simulink library "sm_rollerV_lib_underc_i1u2l7"  (R2026a)
settings: Solver=VariableStepAuto
undefined symbols (not defined in the file): Excv, L1, L2, L3, L4, L5, L6, L7, L8, L9, Left, P1, P2, P3, P4, P5, P6, P7, P8, P9, Right, shoe_w, X, Y, Z
libraries: sm_rollerV_lib_underc_elem x36, sm_lib x27, nesl_utility x20, sm_rollerV_lib_terrain_contact_belem x9, sm_trackV_lib_chain_underc_elem x8, fl_lib x4, sm_trackV_lib_frame_i1u2l7 x2
(part 2 of 3)

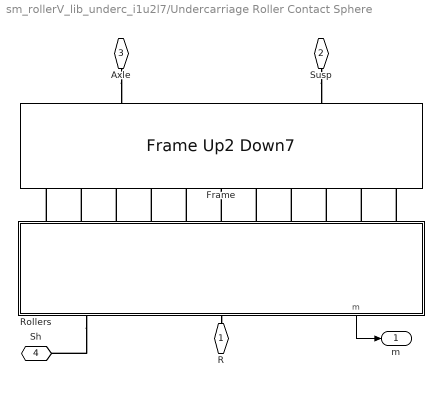
== system sm_rollerV_lib_underc_i1u2l7/Undercarriage Roller Contact Sphere ==
  Frame : sm_trackV_lib_frame_i1u2l7/Frame Up2 Down7  popup_leftOrRight=Right  roller_upper_x=roller_upper_x  roller_lower_x=roller_lower_x  idler_x=idler_x  axle_x=axle_x  roller_upper_y=roller_upper_y  roller_lower_y=roller_lower_y  idler_y=idler_y  axle_y=axle_y  frame_cg_offset=frame_cg_offset  frame_mass=frame_mass  frame_moi=frame_moi  frame_poi=frame_poi  frame_susp_offset=frame_susp_offset
  Rollers : Subsystem  mask(Rollers with Ground Contact (Spheres)){sprk_xc=sprk_xc, sprk_len=sprk_len, sprk_rho=sprk_rho, sprk_clr=sprk_clr, sprk_opc=sprk_opc, sprk_contact_geo_clr=sprk_contact_geo_clr, sprk_contact_geo_opc=sprk_contact_geo_opc, idler_rad=idler_rad, idler_len=idler_len, idler_rho=idler_rho, idler_clr=idler_clr, idler_opc=idler_opc, idler_contact_geo_clr=idler_contact_geo_clr, idler_contact_geo_opc=idler_contact_geo_opc, roller_upper_len=roller_upper_len, roller_upper_rad=roller_upper_rad, roller_upper_rho=roller_upper_rho, roller_upper_clr=roller_upper_clr, roller_upper_opc=roller_upper_opc, roller_upper_contgeo_clr=roller_upper_contgeo_clr, roller_upper_contgeo_opc=roller_upper_contgeo_opc, roller_lower_len=roller_lower_len, roller_lower_rad=roller_lower_rad, roller_lower_rho=roller_lower_rho, roller_lower_clr=roller_lower_clr, roller_lower_opc=roller_lower_opc, roller_lower_contgeo_clr=roller_lower_contgeo_clr, roller_lower_contgeo_opc=roller_lower_contgeo_opc, tensioner_cyl_rad=tensioner_cyl_rad, tensioner_cyl_len=tensioner_cyl_len, tensioner_cyl_rho=tensioner_cyl_rho, tensioner_cyl_clr=tensioner_cyl_clr, tensioner_cyl_opc=tensioner_cyl_opc, tensioner_pist_rad=tensioner_pist_rad, tensioner_pist_len=tensioner_pist_len, tensioner_pist_rho=tensioner_pist_rho, tensioner_pist_clr=tensioner_pist_clr, tensioner_pist_opc=tensioner_pist_opc, tensioner_br_length=tensioner_br_length, tensioner_br_width=tensioner_br_width, tensioner_br_height=tensioner_br_height, tensioner_br_thk=tensioner_br_thk, tensioner_br_rho=tensioner_br_rho, tensioner_br_clr=tensioner_br_clr, tensioner_br_opc=tensioner_br_opc, idler_max_ext=idler_max_ext, sprk_rolling_rad=sprk_rolling_rad, idler_rolling_rad=idler_rolling_rad, roller_lower_rolling_rad=roller_lower_rolling_rad, shoe_w=shoe_w, popup_sense_roller=Actuator Torque}
      mask prompts: sprk_xc "Extrusion Data [x y] (m)"; sprk_len "Length (m)"; sprk_rho "Density (kg/m^3)"; sprk_clr "Color [R G B] (0-1)"; sprk_opc "Opacity (0-1)"; sprk_contact_geo_clr "Color [R G B] (0-1)"; sprk_contact_geo_opc "Opacity (0-1)"; idler_rad "Radius (m)"; idler_len "Length(m)"; idler_rho "Density (kg/m^3)"; idler_clr "Color [R G B] (0-1)"; idler_opc "Opacity (0-1)"; idler_contact_geo_clr "Color [R G B] (0-1)"; idler_contact_geo_opc "Opacity (0-1)"; roller_upper_len "Length (m)"; roller_upper_rad "Radius (m)"; roller_upper_rho "Density (kg/m^3)"; roller_upper_clr "Color [R G B] (0-1)"; roller_upper_opc "Opacity (0-1)"; roller_upper_contgeo_clr "Color [R G B] (0-1)"; roller_upper_contgeo_opc "Opacity (0-1)"; roller_lower_len "Length (m)"; roller_lower_rad "Radius (m)"; roller_lower_rho "Density (kg/m^3)"; roller_lower_clr "Color [R G B] (0-1)"; roller_lower_opc "Opacity (0-1)"; roller_lower_contgeo_clr "Color [R G B] (0-1)"; roller_lower_contgeo_opc "Opacity (0-1)"; tensioner_cyl_rad "Radius (m)"; tensioner_cyl_len "Length (m)"; tensioner_cyl_rho "Density (kg/m^3)"; tensioner_cyl_clr "Color [R G B] (0-1)"; tensioner_cyl_opc "Opacity (0-1)"; tensioner_pist_rad "Radius (m)"; tensioner_pist_len "Length (m)"; tensioner_pist_rho "Density (kg/m^3)"; tensioner_pist_clr "Color [R G B] (0-1)"; tensioner_pist_opc "Opacity (0.1)"; tensioner_br_length "Length (m)"; tensioner_br_width "Width (m)"; tensioner_br_height "Height (m)"; tensioner_br_thk "Thickness (m)"; tensioner_br_rho "Density (kg/m^3)"; tensioner_br_clr "Color [R G B] (0-1)"; tensioner_br_opc "Opacity (0.1)"; idler_max_ext "Max Extension in Track (m)"; sprk_rolling_rad "Sprocket Rolling Radius (m)"; idler_rolling_rad "Idler Rolling Radius (m)"; roller_lower_rolling_rad "Lower Roller Rolling Radius (m)"; shoe_w "Shoe Width (m)"; popup_sense_roller "Roller"
      mask help: Models sprocket, rollers, and idler. Components have sphere contact geometry to enable undercarriage to roll along uneven ground. The sprocket has a 1D rotational mechanical interface to the drivetrain.
      mask init:
      | % Sensing a constraint force can be computationally expensive
      | % Use popup to turn it off if quantity is not needed
      | bh = gcb;
      | rvj_bh = Simulink.findBlocks(bh,'ReferenceBlock','sm_lib/Joints/Revolute Joint');
      | if(strcmp(get_param(bh,'popup_sense_roller'),'Constraint Force'))
      |     SCF = 'on'; STF = 'off';
      |     connectedPort = "fc_out";
      |     senseConstraintTorque = "on";
      |     senseTorqueForce = "off";
      | else
      |     SCF = 'off'; STF = 'on';
      |     connectedPort = "t_out";
      |     senseConstraintTorque = "off";
      |     senseTorqueForce = "on";
      | end
      | 
      | f = Simulink.FindOptions('RegExp',true,'SearchDepth',1);
      | bh_rv = Simulink.findBlocks(bh,'Name','Revolute Lower #*',f);
      | bh_ps = Simulink.findBlocks(bh,'Name','PS-SL Lower #*',f);
      | [~, indrv] = sort(getfullname(bh_rv));
      | [~, indps] = sort(getfullname(bh_ps));
      | bh_rv = bh_rv(indrv);
      | bh_ps = bh_ps(indps);
      | 
      | bh_rvspr = get_param([bh '/Revolute Sprocket'],'Handle');
      | bh_rvidl = get_param([bh '/Revolute Idler'],'Handle');
      | 
      | bh_psspr = get_param([bh '/PS-SL Sprocket'],'Handle');
      | bh_psidl = get_param([bh '/PS-SL Idler'],'Handle');
      | 
      | bh_rv = [bh_rv; bh_rvidl; bh_rvspr];
      | bh_ps = [bh_ps; bh_psidl; bh_psspr];
      | 
      | for i = 1:length(bh_rv)
      |     port_rv = get_param(bh_rv(i),'PortHandles');
      |     port_ps = get_param(bh_ps(i),'PortHandles');
      |     line_rv = get_param(bh_rv(i),'LineHandles');
      | 
      |     if (i==length(bh_rv))
      |         lineInd = 3; % Sprocket joint senses 2 signals
      |     else
      |         lineInd = 2; % All other joints sense 1 signal
      |     end
      |     delete_line(line_rv.RConn(lineInd))
      | 
      |     set_param(bh_rv(i),'SenseConstraintForce',SCF,'SenseTorqueForce',STF);
      |     %port_rv = get_param(bh_rv(1),'PortHandles')
      |     %add_line(bh,port_rv.RConn(lineInd),port_ps.LConn,'autorouting','on');
      |     simscape.addConnection(bh_rv(i), connectedPort, bh_ps(i),'input');
      | end
      mask TypeOptions sprk_xc: Sprocket/sprk_xc
      mask TypeOptions sprk_len: Sprocket/sprk_len
      mask TypeOptions sprk_rho: Sprocket/sprk_rho
      mask TypeOptions sprk_clr: Sprocket/sprk_clr
      mask TypeOptions sprk_opc: Sprocket/sprk_opc
      mask TypeOptions sprk_contact_geo_clr: Sprocket/sprk_contact_geo_clr
      mask TypeOptions sprk_contact_geo_opc: Sprocket/sprk_contact_geo_opc
      mask TypeOptions idler_rad: Idler/idler_rad
      mask TypeOptions idler_len: Idler/idler_len
      mask TypeOptions idler_rho: Idler/idler_rho
      mask TypeOptions idler_clr: Idler/idler_clr
      mask TypeOptions idler_opc: Idler/idler_opc
      mask TypeOptions idler_contact_geo_clr: Idler/idler_contact_geo_clr
      mask TypeOptions idler_contact_geo_opc: Idler/idler_contact_geo_opc
      mask TypeOptions roller_upper_len:
      | Roller
      | Upper 1/roller_upper_len | Roller
      | Upper 2/roller_upper_len
      mask TypeOptions roller_upper_rad:
      | Roller
      | Upper 1/roller_upper_rad | Roller
      | Upper 2/roller_upper_rad
      mask TypeOptions roller_upper_rho:
      | Roller
      | Upper 1/roller_upper_rho | Roller
      | Upper 2/roller_upper_rho
      mask TypeOptions roller_upper_clr:
      | Roller
      | Upper 1/roller_upper_clr | Roller
      | Upper 2/roller_upper_clr
      mask TypeOptions roller_upper_opc:
      | Roller
      | Upper 1/roller_upper_opc | Roller
      | Upper 2/roller_upper_opc
      mask TypeOptions roller_upper_contgeo_clr:
      | Roller
      | Upper 1/roller_upper_contgeo_clr | Roller
      | Upper 2/roller_upper_contgeo_clr
      mask TypeOptions roller_upper_contgeo_opc:
      | Roller
      | Upper 1/roller_upper_contgeo_opc | Roller
      | Upper 2/roller_upper_contgeo_opc
      mask TypeOptions roller_lower_len:
      | Roller
      | Lower 1/roller_lower_len | Roller
      | Lower 2/roller_lower_len | Roller
      | Lower 3/roller_lower_len | Roller
      | Lower 4/roller_lower_len | Roller
      | Lower 5/roller_lower_len | Roller
      | Lower 6/roller_lower_len | Roller
      | Lower 7/roller_lower_len
      mask TypeOptions roller_lower_rad:
      | Roller
      | Lower 1/roller_lower_rad | Roller
      | Lower 2/roller_lower_rad | Roller
      | Lower 3/roller_lower_rad | Roller
      | Lower 4/roller_lower_rad | Roller
      | Lower 5/roller_lower_rad | Roller
      | Lower 6/roller_lower_rad | Roller
      | Lower 7/roller_lower_rad
      mask TypeOptions roller_lower_rho:
      | Roller
      | Lower 1/roller_lower_rho | Roller
      | Lower 2/roller_lower_rho | Roller
      | Lower 3/roller_lower_rho | Roller
      | Lower 4/roller_lower_rho | Roller
      | Lower 5/roller_lower_rho | Roller
      | Lower 6/roller_lower_rho | Roller
      | Lower 7/roller_lower_rho
      mask TypeOptions roller_lower_clr:
      | Roller
      | Lower 1/roller_lower_clr | Roller
      | Lower 2/roller_lower_clr | Roller
      | Lower 3/roller_lower_clr | Roller
      | Lower 4/roller_lower_clr | Roller
      | Lower 5/roller_lower_clr | Roller
      | Lower 6/roller_lower_clr | Roller
      | Lower 7/roller_lower_clr
      mask TypeOptions roller_lower_opc:
      | Roller
      | Lower 1/roller_lower_opc | Roller
      | Lower 2/roller_lower_opc | Roller
      | Lower 3/roller_lower_opc | Roller
      | Lower 4/roller_lower_opc | Roller
      | Lower 5/roller_lower_opc | Roller
      | Lower 6/roller_lower_opc | Roller
      | Lower 7/roller_lower_opc
      mask TypeOptions roller_lower_contgeo_clr:
      | Roller
      | Lower 1/roller_lower_contgeo_clr | Roller
      | Lower 2/roller_lower_contgeo_clr | Roller
      | Lower 3/roller_lower_contgeo_clr | Roller
      | Lower 4/roller_lower_contgeo_clr | Roller
      | Lower 5/roller_lower_contgeo_clr | Roller
      | Lower 6/roller_lower_contgeo_clr | Roller
      | Lower 7/roller_lower_contgeo_clr
      mask TypeOptions roller_lower_contgeo_opc:
      | Roller
      | Lower 1/roller_lower_contgeo_opc | Roller
      | Lower 2/roller_lower_contgeo_opc | Roller
      | Lower 3/roller_lower_contgeo_opc | Roller
      | Lower 4/roller_lower_contgeo_opc | Roller
      | Lower 5/roller_lower_contgeo_opc | Roller
      | Lower 6/roller_lower_contgeo_opc | Roller
      | Lower 7/roller_lower_contgeo_opc
      mask TypeOptions tensioner_cyl_rad:
      | Tensioner
      | Cylinder/cyl_rad
      mask TypeOptions tensioner_cyl_len:
      | Tensioner
      | Cylinder/cyl_len
      mask TypeOptions tensioner_cyl_rho:
      | Tensioner
      | Cylinder/cyl_rho
      mask TypeOptions tensioner_cyl_clr:
      | Tensioner
      | Cylinder/cyl_clr
      mask TypeOptions tensioner_cyl_opc:
      | Tensioner
      | Cylinder/cyl_opc
      mask TypeOptions tensioner_pist_rad:
      | Tensioner
      | Piston/pist_rad
      mask TypeOptions tensioner_pist_len:
      | Tensioner
      | Piston/pist_len
      mask TypeOptions tensioner_pist_rho:
      | Tensioner
      | Piston/pist_rho
      mask TypeOptions tensioner_pist_clr:
      | Tensioner
      | Piston/pist_clr
      mask TypeOptions tensioner_pist_opc:
      | Tensioner
      | Piston/pist_opc
      mask TypeOptions tensioner_br_length:
      | Tensioner
      | Piston/br_length
      mask TypeOptions tensioner_br_width:
      | Tensioner
      | Piston/br_width
      mask TypeOptions tensioner_br_height:
      | Tensioner
      | Piston/br_height
      mask TypeOptions tensioner_br_thk:
      | Tensioner
      | Piston/br_thk
      mask TypeOptions tensioner_br_rho:
      | Tensioner
      | Piston/br_rho
      mask TypeOptions tensioner_br_clr:
      | Tensioner
      | Piston/br_clr
      mask TypeOptions tensioner_br_opc:
      | Tensioner
      | Piston/br_opc
      mask TypeOptions idler_max_ext:
      | Transform
      | Idler Extend/TranslationStandardOffset
      mask TypeOptions sprk_rolling_rad:
      | Constrain
      | Rollers
      | Idler/sprk_rolling_rad | Sprocket/sprk_rolling_rad
      mask TypeOptions idler_rolling_rad:
      | Constrain
      | Rollers
      | Idler/idler_rolling_rad | Idler/idler_rolling_rad
      mask TypeOptions roller_lower_rolling_rad:
      | Constrain
      | Rollers
      | Idler/roller_lower_rolling_rad | Roller
      | Lower 1/roller_lower_rolling_rad | Roller
      | Lower 2/roller_lower_rolling_rad | Roller
      | Lower 3/roller_lower_rolling_rad | Roller
      | Lower 4/roller_lower_rolling_rad | Roller
      | Lower 5/roller_lower_rolling_rad | Roller
      | Lower 6/roller_lower_rolling_rad | Roller
      | Lower 7/roller_lower_rolling_rad
      mask TypeOptions shoe_w:
      | Idler/idler_contact_geo_width | Roller
      | Lower 1/roller_lower_contgeo_width | Roller
      | Lower 2/roller_lower_contgeo_width | Roller
      | Lower 3/roller_lower_contgeo_width | Roller
      | Lower 4/roller_lower_contgeo_width | Roller
      | Lower 5/roller_lower_contgeo_width | Roller
      | Lower 6/roller_lower_contgeo_width | Roller
      | Lower 7/roller_lower_contgeo_width | Sprocket/sprk_contact_geo_w
      mask TypeOptions popup_sense_roller: Constraint Force | Actuator Torque
      mask DialogControl cont_sprk Prompt: Sprocket
      mask DialogControl cont_sprk_solid Prompt: Solid
      mask DialogControl cont_sprk_contact_geo Prompt: Contact Geometry
      mask DialogControl cont_idler Prompt: Idler
      mask DialogControl cont_idler_solid Prompt: Solid
      mask DialogControl cont_idler_contact_geo Prompt: Contact Geometry
      mask DialogControl cont_rollers Prompt: Rollers
      mask DialogControl cont_roller_upper Prompt: Upper
      mask DialogControl cont_roller_upper_contact_geo Prompt: Contact Geometry
      mask DialogControl cont_lower Prompt: Lower
      mask DialogControl cont_lower_contact_geo Prompt: Contact Geometry
      mask DialogControl cont_tensioner Prompt: Tensioner
      mask DialogControl cont_tensioner_cyl Prompt: Cylinder
      mask DialogControl cont_tensioner_pist Prompt: Piston
      mask DialogControl cont_tensioner_brkt Prompt: Bracket
      mask DialogControl cont_tensioner_assy Prompt: Assembly
      mask DialogControl cont_rolling Prompt: Rolling
      mask DialogControl cont_constr_len Prompt: Constraints and Length
      mask DialogControl cont_sensing Prompt: Sensing
      mask Display: image('sm_excv_track_rollerssphere_IMAGE.png');
  R : PMIOPort  Side=Right
  Susp : PMIOPort  Port=2  Side=Right
  Axle : PMIOPort  Port=3  Side=Right
  Sh : PMIOPort  Port=4  Side=Right
  m : Outport
  wires:
  Rollers/1(m) -> m/1
  connections:
  Rollers/RConn1 -- R/RConn1
  Susp/RConn1 -- Frame/LConn1
  Rollers/LConn7 -- Frame/RConn7
  Rollers/LConn5 -- Frame/RConn5
  Rollers/LConn4 -- Frame/RConn4
  Rollers/LConn8 -- Frame/RConn8
  Rollers/LConn10 -- Frame/RConn10
  Rollers/LConn9 -- Frame/RConn9
  Rollers/LConn6 -- Frame/RConn6
  Rollers/LConn1 -- Frame/RConn1
  Rollers/LConn11 -- Frame/RConn11
  Rollers/LConn3 -- Frame/RConn3
  Rollers/LConn2 -- Frame/RConn2
  Rollers/RConn2 -- Sh/RConn1
  Axle/RConn1 -- Frame/LConn2

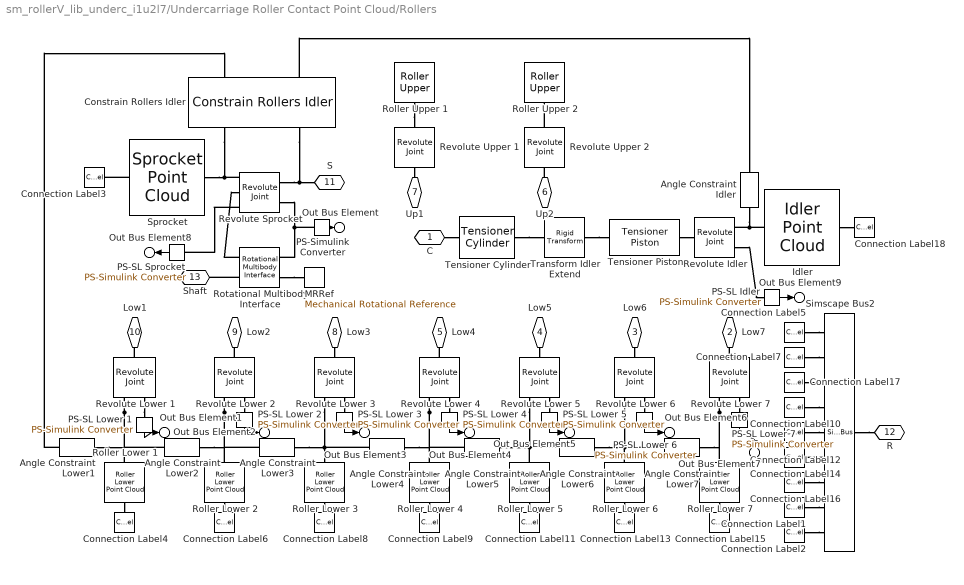
== system sm_rollerV_lib_underc_i1u2l7/Undercarriage Roller Contact Point Cloud/Rollers ==
  Angle Constraint Idler : sm_rollerV_lib_underc_elem/Angle Constraint  SystemSampleTime=-1  VariantActivationTime=update diagram  EmptyChoice=off  PassThrough=off  PassThroughVariantControl=(default)  EmptyChoiceVariantControl=(default)  AllowFlexibleInterface=on  Latency=0  AutoFrameSizeCalculation=off
  Angle Constraint Lower{1..7} (7 alike) : sm_rollerV_lib_underc_elem/Angle Constraint  SystemSampleTime=-1  VariantActivationTime=update diagram  EmptyChoice=off  PassThrough=off  PassThroughVariantControl=(default)  EmptyChoiceVariantControl=(default)  AllowFlexibleInterface=on  Latency=0  AutoFrameSizeCalculation=off
  Connection Label1 : ConnectionLabel  Label=Spr
  Connection Label10 : ConnectionLabel  Label=L4
  Connection Label11 : ConnectionLabel  Label=L5
  Connection Label12 : ConnectionLabel  Label=L5
  Connection Label13 : ConnectionLabel  Label=L6
  Connection Label14 : ConnectionLabel  Label=L6
  Connection Label15 : ConnectionLabel  Label=L7
  Connection Label16 : ConnectionLabel  Label=L7
  Connection Label17 : ConnectionLabel  Label=L3
  Connection Label18 : ConnectionLabel  Label=Idl
  Connection Label2 : ConnectionLabel  Label=Idl
  Connection Label3 : ConnectionLabel  Label=Spr
  Connection Label4 : ConnectionLabel  Label=L1
  Connection Label5 : ConnectionLabel  Label=L1
  Connection Label6 : ConnectionLabel  Label=L2
  Connection Label7 : ConnectionLabel  Label=L2
  Connection Label8 : ConnectionLabel  Label=L3
  Connection Label9 : ConnectionLabel  Label=L4
  Constrain Rollers Idler : sm_rollerV_lib_underc_elem/Constrain Rollers Idler  sprk_rolling_rad=sprk_rolling_rad  roller_lower_rolling_rad=roller_lower_rolling_rad  idler_rolling_rad=idler_rolling_rad
  Idler : sm_rollerV_lib_underc_elem/Idler Point Cloud  idler_rad=idler_rad  idler_len=idler_len  idler_rho=idler_rho  idler_clr=idler_clr  idler_opc=idler_opc  idler_contact_geo_ptcld=idler_contact_geo_ptcld  idler_contact_geo_rad=idler_contact_geo_rad  idler_contact_geo_clr=idler_contact_geo_clr  idler_contact_geo_opc=idler_contact_geo_opc  cyl_rad=idler_rolling_rad  cyl_len=cyl_len  cyl_clr=idler_cyl_clr  cyl_opc=idler_cyl_opc  accMn=accMn  accMx=accMx  acc_clr=acc_clr  acc_opc=acc_opc  lext=lext
  MRRef : fl_lib/Mechanical/Rotational Elements/Mechanical Rotational Reference
  PS-SL Idler : nesl_utility/PS-Simulink Converter  PhysicalDomain=network_engine_domain  SubClassName=ps_output  LeftPortType=input  RightPortType=output  PseudoPeriodic=off  Frequencies=[]  VectorFormat=inherit  Unit=inherit  AffineConversion=off
  PS-SL Lower {1..7} (7 alike) : nesl_utility/PS-Simulink Converter  PhysicalDomain=network_engine_domain  SubClassName=ps_output  LeftPortType=input  RightPortType=output  PseudoPeriodic=off  Frequencies=[]  VectorFormat=inherit  Unit=inherit  AffineConversion=off
  PS-SL Sprocket : nesl_utility/PS-Simulink Converter  PhysicalDomain=network_engine_domain  SubClassName=ps_output  LeftPortType=input  RightPortType=output  PseudoPeriodic=off  Frequencies=[]  VectorFormat=inherit  Unit=inherit  AffineConversion=off
  PS-Simulink Converter : nesl_utility/PS-Simulink Converter  PhysicalDomain=network_engine_domain  SubClassName=ps_output  LeftPortType=input  RightPortType=output  PseudoPeriodic=off  Frequencies=[]  VectorFormat=inherit  Unit=inherit  AffineConversion=off
  Revolute Idler : sm_lib/Joints/Revolute Joint  JointMode=Normal  CompositeWrenchDir=FollowerOnBase  CompositeWrenchFrame=BaseFrame  SenseConstraintForce=off  SenseConstraintTorque=off  SenseTotalForce=off  SenseTotalTorque=off  PositionTargetSpecify=off  PositionTargetPriority=Low  PositionTargetValue=0  PositionTargetValueUnits=deg  VelocityTargetSpecify=off  VelocityTargetPriority=High  VelocityTargetValue=0  VelocityTargetValueUnits=deg/s  EquilibriumPosition=0  EquilibriumPositionUnits=rad  SpringStiffness=0  SpringStiffnessUnits=N*m/rad  DampingCoefficient=0  DampingCoefficientUnits=N*m/(rad/s)  LowerLimitSpecify=off  LowerLimitBound=-90  LowerLimitBoundUnits=deg  LowerLimitStiffness=1e4  LowerLimitStiffnessUnits=N*m/deg  LowerLimitDamping=10  LowerLimitDampingUnits=N*m/(deg/s)  LowerLimitTransitionRegionWidth=0.1  LowerLimitTransitionRegionWidthUnits=deg  UpperLimitSpecify=off  UpperLimitBound=90  UpperLimitBoundUnits=deg  UpperLimitStiffness=1e4  UpperLimitStiffnessUnits=N*m/deg  UpperLimitDamping=10  UpperLimitDampingUnits=N*m/(deg/s)  UpperLimitTransitionRegionWidth=0.1  UpperLimitTransitionRegionWidthUnits=deg  TorqueActuationMode=NoTorque  MotionActuationMode=ComputedMotion  SensePosition=off  SenseVelocity=off  SenseAcceleration=off  SenseTorqueForce=on  SenseLowerLimitTorqueForce=off  SenseUpperLimitTorqueForce=off
  Revolute Lower {1..7} (7 alike) : sm_lib/Joints/Revolute Joint  JointMode=Normal  CompositeWrenchDir=FollowerOnBase  CompositeWrenchFrame=BaseFrame  SenseConstraintForce=off  SenseConstraintTorque=off  SenseTotalForce=off  SenseTotalTorque=off  PositionTargetSpecify=off  PositionTargetPriority=Low  PositionTargetValue=0  PositionTargetValueUnits=deg  VelocityTargetSpecify=off  VelocityTargetPriority=High  VelocityTargetValue=0  VelocityTargetValueUnits=deg/s  EquilibriumPosition=0  EquilibriumPositionUnits=rad  SpringStiffness=0  SpringStiffnessUnits=N*m/rad  DampingCoefficient=0  DampingCoefficientUnits=N*m/(rad/s)  LowerLimitSpecify=off  LowerLimitBound=-90  LowerLimitBoundUnits=deg  LowerLimitStiffness=1e4  LowerLimitStiffnessUnits=N*m/deg  LowerLimitDamping=10  LowerLimitDampingUnits=N*m/(deg/s)  LowerLimitTransitionRegionWidth=0.1  LowerLimitTransitionRegionWidthUnits=deg  UpperLimitSpecify=off  UpperLimitBound=90  UpperLimitBoundUnits=deg  UpperLimitStiffness=1e4  UpperLimitStiffnessUnits=N*m/deg  UpperLimitDamping=10  UpperLimitDampingUnits=N*m/(deg/s)  UpperLimitTransitionRegionWidth=0.1  UpperLimitTransitionRegionWidthUnits=deg  TorqueActuationMode=NoTorque  MotionActuationMode=ComputedMotion  SensePosition=off  SenseVelocity=off  SenseAcceleration=off  SenseTorqueForce=on  SenseLowerLimitTorqueForce=off  SenseUpperLimitTorqueForce=off
  Revolute Sprocket : sm_lib/Joints/Revolute Joint  JointMode=Normal  CompositeWrenchDir=FollowerOnBase  CompositeWrenchFrame=BaseFrame  SenseConstraintForce=off  SenseConstraintTorque=off  SenseTotalForce=off  SenseTotalTorque=off  PositionTargetSpecify=off  PositionTargetPriority=Low  PositionTargetValue=0  PositionTargetValueUnits=deg  VelocityTargetSpecify=off  VelocityTargetPriority=High  VelocityTargetValue=0  VelocityTargetValueUnits=deg/s  EquilibriumPosition=0  EquilibriumPositionUnits=rad  SpringStiffness=0  SpringStiffnessUnits=N*m/rad  DampingCoefficient=0  DampingCoefficientUnits=N*m/(rad/s)  LowerLimitSpecify=off  LowerLimitBound=-90  LowerLimitBoundUnits=deg  LowerLimitStiffness=1e4  LowerLimitStiffnessUnits=N*m/deg  LowerLimitDamping=10  LowerLimitDampingUnits=N*m/(deg/s)  LowerLimitTransitionRegionWidth=0.1  LowerLimitTransitionRegionWidthUnits=deg  UpperLimitSpecify=off  UpperLimitBound=90  UpperLimitBoundUnits=deg  UpperLimitStiffness=1e4  UpperLimitStiffnessUnits=N*m/deg  UpperLimitDamping=10  UpperLimitDampingUnits=N*m/(deg/s)  UpperLimitTransitionRegionWidth=0.1  UpperLimitTransitionRegionWidthUnits=deg  TorqueActuationMode=InputTorque  MotionActuationMode=ComputedMotion  SensePosition=off  SenseVelocity=on  SenseAcceleration=off  SenseTorqueForce=on  SenseLowerLimitTorqueForce=off  SenseUpperLimitTorqueForce=off
  Revolute Upper 1 : sm_lib/Joints/Revolute Joint  JointMode=Normal  CompositeWrenchDir=FollowerOnBase  CompositeWrenchFrame=BaseFrame  SenseConstraintForce=off  SenseConstraintTorque=off  SenseTotalForce=off  SenseTotalTorque=off  PositionTargetSpecify=off  PositionTargetPriority=Low  PositionTargetValue=0  PositionTargetValueUnits=deg  VelocityTargetSpecify=off  VelocityTargetPriority=High  VelocityTargetValue=0  VelocityTargetValueUnits=deg/s  EquilibriumPosition=0  EquilibriumPositionUnits=rad  SpringStiffness=0  SpringStiffnessUnits=N*m/rad  DampingCoefficient=0  DampingCoefficientUnits=N*m/(rad/s)  LowerLimitSpecify=off  LowerLimitBound=-90  LowerLimitBoundUnits=deg  LowerLimitStiffness=1e4  LowerLimitStiffnessUnits=N*m/deg  LowerLimitDamping=10  LowerLimitDampingUnits=N*m/(deg/s)  LowerLimitTransitionRegionWidth=0.1  LowerLimitTransitionRegionWidthUnits=deg  UpperLimitSpecify=off  UpperLimitBound=90  UpperLimitBoundUnits=deg  UpperLimitStiffness=1e4  UpperLimitStiffnessUnits=N*m/deg  UpperLimitDamping=10  UpperLimitDampingUnits=N*m/(deg/s)  UpperLimitTransitionRegionWidth=0.1  UpperLimitTransitionRegionWidthUnits=deg  TorqueActuationMode=NoTorque  MotionActuationMode=ComputedMotion  SensePosition=off  SenseVelocity=off  SenseAcceleration=off  SenseTorqueForce=off  SenseLowerLimitTorqueForce=off  SenseUpperLimitTorqueForce=off
  Revolute Upper 2 : sm_lib/Joints/Revolute Joint  JointMode=Normal  CompositeWrenchDir=FollowerOnBase  CompositeWrenchFrame=BaseFrame  SenseConstraintForce=off  SenseConstraintTorque=off  SenseTotalForce=off  SenseTotalTorque=off  PositionTargetSpecify=off  PositionTargetPriority=Low  PositionTargetValue=0  PositionTargetValueUnits=deg  VelocityTargetSpecify=off  VelocityTargetPriority=High  VelocityTargetValue=0  VelocityTargetValueUnits=deg/s  EquilibriumPosition=0  EquilibriumPositionUnits=rad  SpringStiffness=0  SpringStiffnessUnits=N*m/rad  DampingCoefficient=0  DampingCoefficientUnits=N*m/(rad/s)  LowerLimitSpecify=off  LowerLimitBound=-90  LowerLimitBoundUnits=deg  LowerLimitStiffness=1e4  LowerLimitStiffnessUnits=N*m/deg  LowerLimitDamping=10  LowerLimitDampingUnits=N*m/(deg/s)  LowerLimitTransitionRegionWidth=0.1  LowerLimitTransitionRegionWidthUnits=deg  UpperLimitSpecify=off  UpperLimitBound=90  UpperLimitBoundUnits=deg  UpperLimitStiffness=1e4  UpperLimitStiffnessUnits=N*m/deg  UpperLimitDamping=10  UpperLimitDampingUnits=N*m/(deg/s)  UpperLimitTransitionRegionWidth=0.1  UpperLimitTransitionRegionWidthUnits=deg  TorqueActuationMode=NoTorque  MotionActuationMode=ComputedMotion  SensePosition=off  SenseVelocity=off  SenseAcceleration=off  SenseTorqueForce=off  SenseLowerLimitTorqueForce=off  SenseUpperLimitTorqueForce=off
  Roller Lower {1..7} (7 alike) : sm_rollerV_lib_underc_elem/Roller Lower Point Cloud  roller_lower_rad=roller_lower_rad  roller_lower_len=roller_lower_len  roller_lower_rho=roller_lower_rho  roller_lower_clr=roller_lower_clr  roller_lower_opc=roller_lower_opc  roller_lower_contgeo_ptcld=roller_lower_contgeo_ptcld  roller_lower_contgeo_rad=roller_lower_contgeo_rad  roller_lower_contgeo_clr=roller_lower_contgeo_clr  roller_lower_contgeo_opc=roller_lower_contgeo_opc  cyl_rad=roller_lower_rolling_rad  cyl_len=cyl_len  cyl_clr=roller_cyl_clr  cyl_opc=roller_cyl_opc  accMn=accMn  accMx=accMx  acc_clr=acc_clr  acc_opc=acc_opc  lext=lext
      settings: LibrarySourceBlock=sm_chain_drive_lib/Pulley_Bot
  Roller Upper 1 : sm_trackV_lib_chain_underc_elem/Roller Upper  roller_upper_rad=roller_upper_rad  roller_upper_len=roller_upper_len  roller_upper_rho=roller_upper_rho  roller_upper_clr=roller_upper_clr  roller_upper_opc=roller_upper_opc  roller_upper_contgeo_clr=roller_upper_contgeo_clr  roller_upper_contgeo_opc=roller_upper_contgeo_opc
      settings: LibrarySourceBlock=sm_chain_drive_lib/Pulley_Top
  Roller Upper 2 : sm_trackV_lib_chain_underc_elem/Roller Upper  roller_upper_rad=roller_upper_rad  roller_upper_len=roller_upper_len  roller_upper_rho=roller_upper_rho  roller_upper_clr=roller_upper_clr  roller_upper_opc=roller_upper_opc  roller_upper_contgeo_clr=roller_upper_contgeo_clr  roller_upper_contgeo_opc=roller_upper_contgeo_opc
      settings: LibrarySourceBlock=sm_chain_drive_lib/Pulley_Top
  Rotational Multibody Interface : fl_lib/Mechanical/Multibody Interfaces/Rotational Multibody Interface
  Simscape Bus2 : SimscapeBus  HierarchyStrings=P1;P2;P3;P4;P5;P6;P7;P8;P9  ConnectionType=Bus: CBO_Roller9
  Sprocket : sm_rollerV_lib_underc_elem/Sprocket Point Cloud  sprk_xc=sprk_xc  sprk_len=sprk_len  sprk_rho=sprk_rho  sprk_clr=sprk_clr  sprk_opc=sprk_opc  sprk_contact_geo_ptcld=sprk_contact_geo_ptcld  sprk_contact_geo_rad=sprk_contact_geo_rad  sprk_contact_geo_clr=sprk_contact_geo_clr  sprk_contact_geo_opc=sprk_contact_geo_opc  cyl_rad=sprk_rolling_rad  cyl_len=cyl_len  cyl_clr=sprocket_cyl_clr  cyl_opc=sprocket_cyl_opc  accMn=accMn  accMx=accMx  acc_clr=acc_clr  acc_opc=acc_opc  lext=lext
  Tensioner Cylinder : sm_trackV_lib_chain_underc_elem/Tensioner Cylinder  cyl_rad=tensioner_cyl_rad  cyl_len=tensioner_cyl_len  cyl_rho=tensioner_cyl_rho  cyl_clr=tensioner_cyl_clr  cyl_opc=tensioner_cyl_opc  brk_len=Excv.Idler.Tensioner.bracket.len  brk_thk=Excv.Idler.Tensioner.bracket.thk  pist_len=Excv.Idler.Tensioner.piston.len
      settings: LibrarySourceBlock=sm_chain_drive_lib/Idler_Housing
  Tensioner Piston : sm_trackV_lib_chain_underc_elem/Tensioner Piston  pist_rad=tensioner_pist_rad  pist_len=tensioner_pist_len  pist_rho=tensioner_pist_rho  pist_clr=tensioner_pist_clr  pist_opc=tensioner_pist_opc  br_height=tensioner_br_height  br_length=tensioner_br_length  br_width=tensioner_br_width  br_rho=tensioner_br_rho  br_thk=tensioner_br_thk  br_clr=tensioner_br_clr  br_opc=tensioner_br_opc
      settings: LibrarySourceBlock=sm_chain_drive_lib/ldler_Damper
  Transform Idler Extend : sm_lib/Frames and Transforms/Rigid Transform  RotationMethod=None  FollAlignAxisA=+X  BaseAlignAxisA=+Y  FollAlignAxisB=+Y  BaseAlignAxisB=+Z  RotationStandardAxis=+Z  RotationAngle=0.1  RotationAngleUnits=deg  RotationArbitraryAxis=[0 0 1]  RotationSequenceAxes=FollowerAxes  RotationSequence=XYX  RotationSequenceAngles=[0 0 0]  RotationSequenceAnglesUnits=deg  RotationMatrix=[1 0 0; 0 1 0; 0 0 1]  Quaternion=[1 0 0 0]  TranslationMethod=StandardAxis  TranslationCartesianOffset=[0 0 0]  TranslationCartesianOffsetUnits=m  TranslationStandardAxis=+Z  TranslationStandardOffset=idler_max_ext  TranslationStandardOffsetUnits=m  TranslationROffset=0  TranslationROffsetUnits=m  TranslationThetaOffset=0  TranslationThetaOffsetUnits=deg  TranslationZOffset=0  TranslationZOffsetUnits=m
  C : PMIOPort  Side=Left
  Low7 : PMIOPort  Port=2  Side=Left
  Low6 : PMIOPort  Port=3  Side=Left
  Low5 : PMIOPort  Port=4  Side=Left
  Low4 : PMIOPort  Port=5  Side=Left
  Up2 : PMIOPort  Port=6  Side=Left
  Up1 : PMIOPort  Port=7  Side=Left
  Low3 : PMIOPort  Port=8  Side=Left
  Low2 : PMIOPort  Port=9  Side=Left
  Low1 : PMIOPort  Port=10  Side=Left
  S : PMIOPort  Port=11  Side=Left
  R : PMIOPort  Port=12  Side=Right
  Shaft : PMIOPort  Port=13  Side=Right
  Out Bus Element : Outport  PortName=m  Element=tSprk
  Out Bus Element1 : Outport  PortName=m  Element=RL1
  Out Bus Element2 : Outport  PortName=m  Element=RL2
  Out Bus Element3 : Outport  PortName=m  Element=RL3
  Out Bus Element4 : Outport  PortName=m  Element=RL4
  Out Bus Element5 : Outport  PortName=m  Element=RL5
  Out Bus Element6 : Outport  PortName=m  Element=RL6
  Out Bus Element7 : Outport  PortName=m  Element=RL7
  Out Bus Element8 : Outport  PortName=m  Element=XSprk
  Out Bus Element9 : Outport  PortName=m  Element=XIdlerF
  wires:
  PS-SL Lower 7/1 -> Out Bus Element7/1
  PS-SL Lower 6/1 -> Out Bus Element6/1
  PS-SL Lower 5/1 -> Out Bus Element5/1
  PS-SL Lower 4/1 -> Out Bus Element4/1
  PS-SL Lower 3/1 -> Out Bus Element3/1
  PS-SL Lower 2/1 -> Out Bus Element2/1
  PS-SL Lower 1/1 -> Out Bus Element1/1
  PS-Simulink Converter/1 -> Out Bus Element/1
  PS-SL Sprocket/1 -> Out Bus Element8/1
  PS-SL Idler/1 -> Out Bus Element9/1
  connections:
  Connection Label2/LConn1 -- Simscape Bus2/LConn9
  Connection Label1/LConn1 -- Simscape Bus2/LConn8
  Angle Constraint Lower1/LConn1 -- Constrain Rollers Idler/RConn1
  Constrain Rollers Idler/RConn2 -- Angle Constraint Idler/LConn1
  Tensioner Cylinder/RConn1 -- Transform Idler Extend/LConn1
  C/RConn1 -- Tensioner Cylinder/LConn1
  Transform Idler Extend/RConn1 -- Tensioner Piston/LConn1
  Idler/RConn1 -- Connection Label18/LConn1
  Roller Lower 6/RConn1 -- Connection Label13/LConn1
  Roller Lower 2/RConn1 -- Connection Label6/LConn1
  Revolute Upper 1/LConn1 -- Up1/RConn1
  Roller Lower 4/RConn1 -- Connection Label9/LConn1
  Roller Lower 7/RConn1 -- Connection Label15/LConn1
  Revolute Lower 6/RConn1 -- Angle Constraint Lower7/LConn1 -- Angle Constraint Lower6/RConn1 -- Roller Lower 6/LConn1
  Roller Lower 3/RConn1 -- Connection Label8/LConn1
  S/RConn1 -- Constrain Rollers Idler/LConn2 -- Revolute Sprocket/LConn1
  Roller Lower 5/RConn1 -- Connection Label11/LConn1
  Simscape Bus2/RConn1 -- R/RConn1
  Revolute Idler/RConn1 -- Idler/LConn1 -- Angle Constraint Idler/RConn1
  Sprocket/LConn1 -- Constrain Rollers Idler/LConn1 -- Revolute Sprocket/RConn1
  Revolute Lower 5/RConn1 -- Angle Constraint Lower6/LConn1 -- Angle Constraint Lower5/RConn1 -- Roller Lower 5/LConn1
  Revolute Upper 2/RConn1 -- Roller Upper 2/LConn1
  Revolute Lower 2/LConn1 -- Low2/RConn1
  Tensioner Piston/RConn1 -- Revolute Idler/LConn1
  Sprocket/RConn1 -- Connection Label3/LConn1
  Roller Lower 1/RConn1 -- Connection Label4/LConn1
  Revolute Lower 4/LConn1 -- Low4/RConn1
  Revolute Lower 3/RConn1 -- Angle Constraint Lower4/LConn1 -- Angle Constraint Lower3/RConn1 -- Roller Lower 3/LConn1
  Revolute Lower 7/LConn1 -- Low7/RConn1
  Revolute Lower 1/LConn1 -- Low1/RConn1
  Connection Label10/LConn1 -- Simscape Bus2/LConn4
  Connection Label17/LConn1 -- Simscape Bus2/LConn3
  Connection Label7/LConn1 -- Simscape Bus2/LConn2
  Connection Label16/LConn1 -- Simscape Bus2/LConn7
  Simscape Bus2/LConn6 -- Connection Label14/LConn1
  Connection Label12/LConn1 -- Simscape Bus2/LConn5
  Connection Label5/LConn1 -- Simscape Bus2/LConn1
  Low5/RConn1 -- Revolute Lower 5/LConn1
  Revolute Lower 2/RConn1 -- Angle Constraint Lower3/LConn1 -- Angle Constraint Lower2/RConn1 -- Roller Lower 2/LConn1
  Low3/RConn1 -- Revolute Lower 3/LConn1
  Revolute Lower 7/RConn1 -- Angle Constraint Lower7/RConn1 -- Roller Lower 7/LConn1
  Revolute Lower 1/RConn1 -- Angle Constraint Lower1/RConn1 -- Angle Constraint Lower2/LConn1 -- Roller Lower 1/LConn1
  Revolute Lower 4/RConn1 -- Angle Constraint Lower4/RConn1 -- Angle Constraint Lower5/LConn1 -- Roller Lower 4/LConn1
  Low6/RConn1 -- Revolute Lower 6/LConn1
  Roller Upper 1/LConn1 -- Revolute Upper 1/RConn1
  Up2/RConn1 -- Revolute Upper 2/LConn1
  Revolute Sprocket/LConn2 -- Rotational Multibody Interface/LConn1 -- PS-Simulink Converter/LConn1
  Rotational Multibody Interface/RConn1 -- Revolute Sprocket/RConn2
  Rotational Multibody Interface/RConn2 -- Shaft/RConn1
  Rotational Multibody Interface/LConn2 -- MRRef/LConn1
  Revolute Lower 1/RConn2 -- PS-SL Lower 1/LConn1
  Revolute Lower 2/RConn2 -- PS-SL Lower 2/LConn1
  Revolute Lower 3/RConn2 -- PS-SL Lower 3/LConn1
  Revolute Lower 4/RConn2 -- PS-SL Lower 4/LConn1
  Revolute Lower 5/RConn2 -- PS-SL Lower 5/LConn1
  Revolute Lower 6/RConn2 -- PS-SL Lower 6/LConn1
  Revolute Lower 7/RConn2 -- PS-SL Lower 7/LConn1
  Revolute Idler/RConn2 -- PS-SL Idler/LConn1
  Revolute Sprocket/RConn3 -- PS-SL Sprocket/LConn1
